simulink model "vehicle_body_model"  (R2024b)
settings: Solver=ode23tb  StartTime=0.0  StopTime=300.0  RelTol=1e-3
libraries: SignalEditorBlockLib x1, slpidlib x1
settings Model: Creator=this pc  LastModifiedBy=this pc

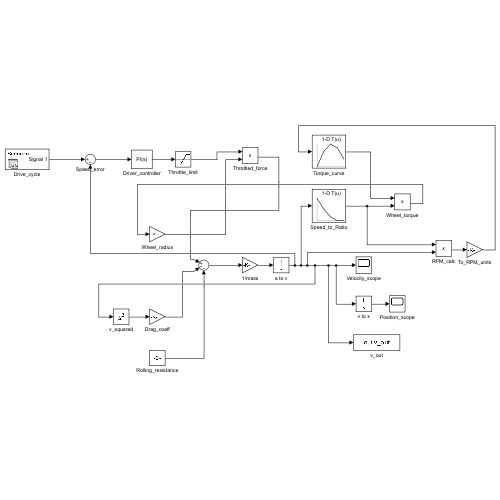
[thumbnail: Simulink's stored preview of the top-level diagram]
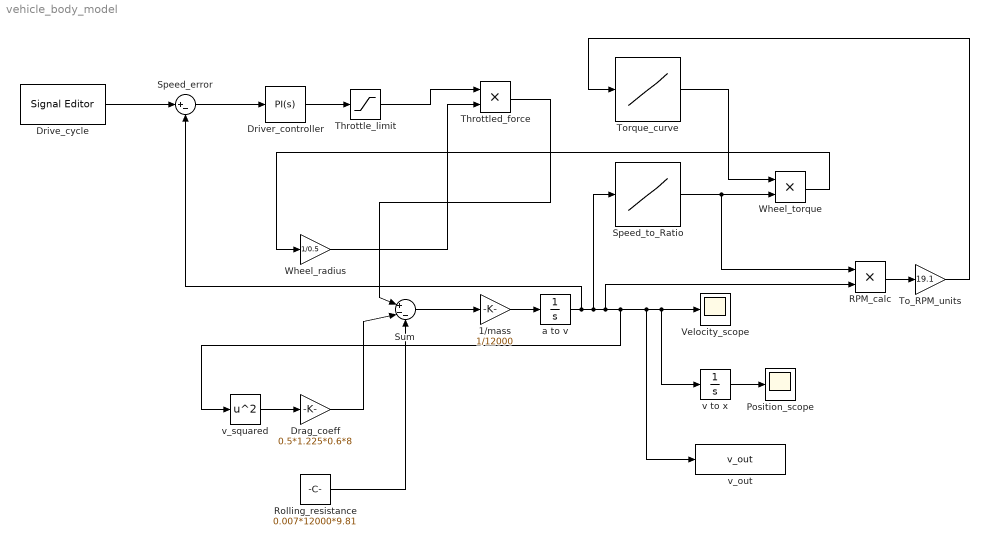
== system vehicle_body_model ==
  1/mass : Gain  Gain=1/12000
  Drag_coeff : Gain  Gain=0.5*1.225*0.6*8
  Drive_cycle : SignalEditorBlockLib/Signal Editor  FileName=untitled.mat  ActiveScenario=Scenario  ActiveSignal=Signal 1  IsBus=off  OutputBusObjectStr=Bus: BusObject  SampleTime=0  Interpolate=off  ZeroCross=off  OutputAfterFinalValue=Setting to zero  Unit=inherit  PreserveSignalName=on  ApplySigPropsToAllScenarios=on  ApplySigPropsToAllSignals=off
  Driver_controller : slpidlib/PID Controller  Controller=PI  Form=Parallel  TimeDomain=Continuous-time  UseExternalTs=off  SampleTime=-1  IntegratorMethod=Forward Euler  FilterMethod=Forward Euler  ControllerParametersSource=internal  P=5000  I=500  UseKiTs=off  D=0  UseExternalDerivativeSource=off  N=100  UseFilter=on  TunerSelectOption=Transfer Function Based (PID Tuner App)  InitialConditionSource=internal  InitialConditionForIntegrator=0  InitialConditionForFilter=0  DifferentiatorICPrevScaledInput=0  ExternalReset=none  TrackingMode=off  Kt=1  LimitOutput=off  SatLimitsSource=internal  UpperSaturationLimit=inf  LowerSaturationLimit=-inf  LinearizeAsGain=on  AntiWindupMode=none  Kb=1  LimitIntegrator=off  UpperIntegratorSaturationLimit=inf  LowerIntegratorSaturationLimit=-inf  POutMin=[]  POutMax=[]  IOutMin=[]  IOutMax=[]  DOutMin=[]  DOutMax=[]  NOutMin=[]  NOutMax=[]  SumOutMin=[]  SumOutMax=[]  SaturationOutMin=[]  SaturationOutMax=[]  PParamMin=[]  PParamMax=[]  IParamMin=[]  IParamMax=[]  DParamMin=[]  DParamMax=[]  NParamMin=[]  NParamMax=[]  KbParamMin=[]  KbParamMax=[]  KtParamMin=[]  KtParamMax=[]  KbOutMin=[]  KbOutMax=[]  KtOutMin=[]  KtOutMax=[]  IntegratorOutMin=[]  IntegratorOutMax=[]  FilterOutMin=[]  FilterOutMax=[]  SumI1OutMin=[]  SumI1OutMax=[]  SumI2OutMin=[]  SumI2OutMax=[]  SumI3OutMin=[]  SumI3OutMax=[]  SumI4OutMin=[]  SumI4OutMax=[]  SumDOutMin=[]  SumDOutMax=[]  DifferentiatorOutMin=[]  DifferentiatorOutMax=[]  FilterDiffOutCoefMin=[]  FilterDiffOutCoefMax=[]  ReciprocalOutMin=[]  ReciprocalOutMax=[]  SumDenOutMin=[]  SumDenOutMax=[]  SumNumOutMin=[]  SumNumOutMax=[]  DivideOutMin=[]  DivideOutMax=[]  UdiffTsProdOutMin=[]  UdiffTsProdOutMax=[]  NTsProdOutMin=[]  NTsProdOutMax=[]  UintegralTsProdOutMin=[]  UintegralTsProdOutMax=[]  UngainTsProdOutMin=[]  UngainTsProdOutMax=[]  ClampingZeroOutDataTypeStr=Inherit: Inherit via back propagation  ClampingZeroOutMin=[]  ClampingZeroOutMax=[]  FilterDenConstantOutDataTypeStr=Inherit: Inherit via back propagation  FilterDenConstantOutMin=[]  FilterDenConstantOutMax=[]  PCopyOutDataTypeStr=Inherit: Inherit via back propagation  PCopyOutMin=[]  PCopyOutMax=[]  NCopyOutDataTypeStr=Inherit: Inherit via back propagation  NCopyOutMin=[]  NCopyOutMax=[]  IntegratorContinuousStateAttributes=''  IntegratorStateMustResolveToSignalObject=off  IntegratorRTWStateStorageClass=Auto  FilterContinuousStateAttributes=''  FilterStateMustResolveToSignalObject=off  FilterRTWStateStorageClass=Auto  ParallelPVariant=InternalParameters  IdealPVariant=Disabled  IVariant=InternalParameters  DVariant=Disabled  IntegratorVariant=Continuous  SatVariant=Disabled  AWVariant=Passthrough  PCopyVariant=Disabled  TRVariant=Disabled  FdbkBlocksVariant=Forward  IdealPFdbkVariant=Disabled  SatFdbkVariant=Disabled  DerivativeFilterVariant=Disabled  NVariant=Disabled  NCopyVariant=Disabled_SignalSpec  FilterICVariant=Disabled  IntegratorICVariant=InternalICs  ExternalResetVariant=Disabled  TRSumVariant=Passthrough  SumFdbkVariant=Disabled  SumVariant=Sum_PI  TsampFilterVariant=InternalTs  TsampNgainVariant=Passthrough  TsampIntegralVariant=Disabled_SignalSpec  ExternalSaturationOutDataTypeStr=Inherit: Same as second input  DerivativeSourceVariant=Disabled  PreIntVariant=InternalPreInt
  Position_scope : Scope
  RPM_calc : Product
  Rolling_resistance : Constant  Value=0.007*12000*9.81
  Speed_error : Sum  Inputs=|+-
  Speed_to_Ratio : Lookup_n-D  NumberOfTableDimensions=1  BreakpointsForDimension1=[0 5 10 15 20]  Table=[32 20 12 8 8]  ExtrapMethod=Clip  InternalRulePriority=Speed  RndMeth=Simplest
  Sum : Sum  Inputs=|+--
  Throttle_limit : Saturate  UpperLimit=1  LowerLimit=0
  Throttled_force : Product
  To_RPM_units : Gain  Gain=19.1
  Torque_curve : Lookup_n-D  NumberOfTableDimensions=1  BreakpointsForDimension1=[800 1200 1600 2000 2400]  Table=[600 1400 1800 1600 1000]  ExtrapMethod=Clip  InternalRulePriority=Speed  RndMeth=Simplest
  Velocity_scope : Scope
  Wheel_radius : Gain  Gain=1/0.5
  Wheel_torque : Product
  a to v : Integrator
  v to x : Integrator
  v_out : ToWorkspace  VariableName=v_out  SampleTime=-1
  v_squared : Math  Operator=square
  wires:
  Sum/1 -> 1/mass/1
  1/mass/1 -> a to v/1
  a to v/1 -> Speed_error/2, RPM_calc/2, Velocity_scope/1, v to x/1, v_out/1, v_squared/1, Speed_to_Ratio/1
  v to x/1 -> Position_scope/1
  v_squared/1 -> Drag_coeff/1
  Drag_coeff/1 -> Sum/2
  Rolling_resistance/1 -> Sum/3
  Wheel_radius/1 -> Throttled_force/2
  RPM_calc/1 -> To_RPM_units/1
  To_RPM_units/1 -> Torque_curve/1
  Torque_curve/1 -> Wheel_torque/1
  Speed_to_Ratio/1 -> Wheel_torque/2, RPM_calc/1
  Wheel_torque/1 -> Wheel_radius/1
  Drive_cycle/1 -> Speed_error/1
  Speed_error/1 -> Driver_controller/1
  Driver_controller/1 -> Throttle_limit/1
  Throttle_limit/1 -> Throttled_force/1
  Throttled_force/1 -> Sum/1
